simulink model "cell_EC_model"  (R2024a)
settings: Solver=VariableStepAuto  StartTime=0.0  StopTime=stop_time  FixedStep=0.5  MaxStep=.1  RelTol=1e-3
values from neighbouring files (symbols this model uses):
  C1c = data(2:end, 2:end)    [plot_RC_params.m]    (also in run_cell_sim.m)
  C1d = data(2:end, 2:end)    [plot_RC_params.m]    (also in run_cell_sim.m)
  C2c = data(2:end, 2:end)    [plot_RC_params.m]    (also in run_cell_sim.m)
  C2d = data(2:end, 2:end)    [plot_RC_params.m]    (also in run_cell_sim.m)
  C3c = data(2:end, 2:end)    [plot_RC_params.m]    (also in run_cell_sim.m)
  C3d = data(2:end, 2:end)    [plot_RC_params.m]    (also in run_cell_sim.m)
  capacity = 115.8    [extract_R0.m]    (also in identify_pulses.m; optimise_RC_parameters.m = params(7); run_cell_sim.m)
  OCV_SOC = data(2:end, 1)    [run_cell_sim.m]
  OCV_T = data(1, 2:end)    [run_cell_sim.m]
  OCV_V = data(2:end, 2:end)    [run_cell_sim.m]
  R0c = data(2:end, 2:end)    [plot_RC_params.m]    (also in run_cell_sim.m)
  R0d = data(2:end, 2:end)    [plot_RC_params.m]    (also in run_cell_sim.m)
  R1c = data(2:end, 2:end)    [plot_RC_params.m]    (also in run_cell_sim.m)
  R1d = data(2:end, 2:end)    [plot_RC_params.m]    (also in run_cell_sim.m)
  R2c = data(2:end, 2:end)    [plot_RC_params.m]    (also in run_cell_sim.m)
  R2d = data(2:end, 2:end)    [plot_RC_params.m]    (also in run_cell_sim.m)
  R3c = data(2:end, 2:end)    [plot_RC_params.m]    (also in run_cell_sim.m)
  R3d = data(2:end, 2:end)    [plot_RC_params.m]    (also in run_cell_sim.m)
  RC_SOC = data(1, 2:end)    [plot_RC_params.m]    (also in run_cell_sim.m)
  RC_T = data(2:end, 1)    [plot_RC_params.m]    (also in run_cell_sim.m)
  soc_in = interp1(OCV.V(:, find(OCV.T == temperature)), OCV.SOC, actual_voltage_full.Data(1), "linear", 'extrap')    [optimise_RC_parameters.m]    (also in run_cell_sim.m = 1)
libraries: nesl_utility x13, fl_lib x9, ee_lib x3
settings Model: Creator=mmackenzie  LastModifiedBy=mmackenzie
settings OptimizationCC: ReuseModelBlockBuffer=off
settings RTWCC: GPUComputeCapability=3.5

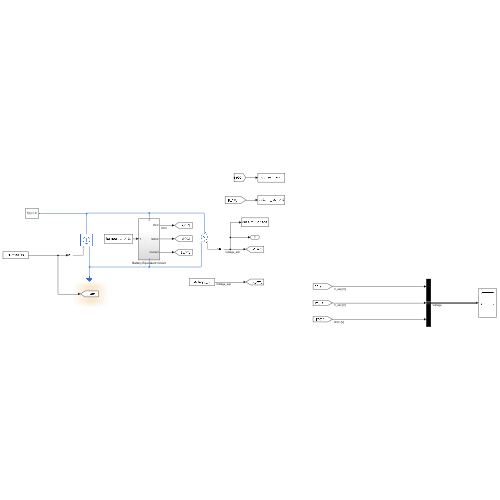
[thumbnail: Simulink's stored preview of the top-level diagram]
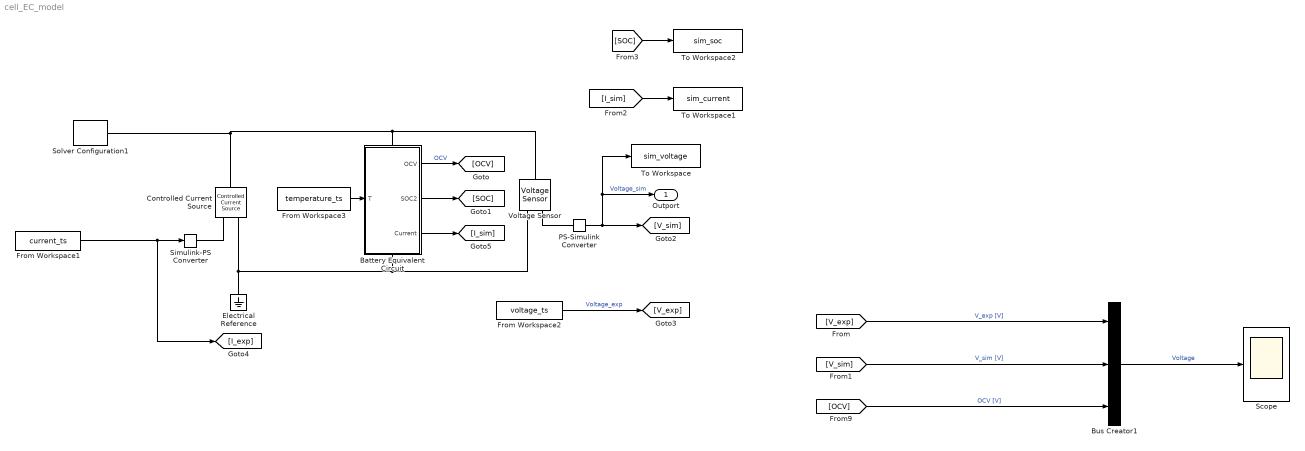
== system cell_EC_model ==
  Battery Equivalent Circuit : Subsystem
      settings: PortSchema="{\"entries\":[{\"content\":{\"sides\":[{\"content\":{\"connectorIds\":[\"In1\"]},\"type\":\"ConnectorPlacement.EquallySpacedRectSide\",\"uuid\":\"397b6d9d-31ba-4533-8816-c8a956765ed5\"},{\"content\":{\"connectorIds\":[\"Out1\",\"Out2\",\"Out3\"],\"side\":\"RIGHT\"},\"type\":\"ConnectorPlacement.EquallySpacedRectSide\",\"uuid\":\"178b2ca9-d2d9-4380-91aa-f4497cccdf4f\"},{\"content\":{\"connectorIds\":[\"LConn1\"],\"side\":\"TOP\"},\"type\":\"ConnectorPlacement.EquallySpacedRectSide\",\"uuid\":\"4710d0ae-2920-4204-9cef-cbb5eb77e7ed\"},{\"content\":{\"connectorIds\":[\"RConn1\"],\"side\":\"BOTTOM\"},\"type\":\"ConnectorPlacement.EquallySpacedRectSide\",\"uuid\":\"673921ba-ed04-43cc-8806-353dbfb62c12\"}]},\"type\":\"ConnectorPlacement.EquallySpacedConnector\",\"uuid\":\"77ff7300-8565-4430-8966-d92537bdab4b\"}],\"packageUris\":[\"http://schema.mathworks.com/mf0/Connector/R2020b\"],\"version\":\"1.0\"}"
  Bus Creator1 : BusCreator  Inputs=3
  Controlled Current Source : fl_lib/Electrical/Electrical Sources/Controlled Current Source
  Electrical Reference : fl_lib/Electrical/Electrical Elements/Electrical Reference
  From Workspace1 : FromWorkspace  VariableName=current_ts  SampleTime=-1
  From Workspace2 : FromWorkspace  VariableName=voltage_ts  SampleTime=-1
  From Workspace3 : FromWorkspace  VariableName=temperature_ts  SampleTime=-1
  PS-Simulink Converter : nesl_utility/PS-Simulink Converter  PhysicalDomain=network_engine_domain  SubClassName=ps_output  LeftPortType=input  RightPortType=output  PseudoPeriodic=off  Frequencies=[]  VectorFormat=inherit  Unit=inherit  AffineConversion=off
  Scope : Scope
  Simulink-PS Converter : nesl_utility/Simulink-PS Converter  PhysicalDomain=network_engine_domain  SubClassName=ps_input  LeftPortType=input  RightPortType=output  PseudoPeriodic=off  Frequencies=[]  NoiseDistribution=none  NoiseParameters=[]  Unit=1  AffineConversion=off  FilteringAndDerivatives=provide  SimscapeFilterOrder=1  InputFilterTimeConstant=0.001  UdotUserProvided=0
  Solver Configuration1 : nesl_utility/Solver Configuration  PhysicalDomain=network_engine_domain  SubClassName=solver  LeftPortType=input  RightPortType=generic  Tones=[]  Harmonics=[]  SimulateNoise=off  Profile=off  UseLocalSampling=off  EnableSwitchedLinearOptims=on  FrequencyDomain=off  UseCCode=off  RelTol=0.001  AbsTol=0.001  MinStep=1e-09  ToWorkspace=off  RevertToSquareIcSolve=off  NumHomotopyIterations=100  PhasorMode=off  PhasorModeNumHarmonics=1  ConsistencySolver=NEWTON_FTOL  IndexReductionMethod=DerivativeReplacement  DoDC=off  ResidualTolerance=1e-09  ConsistencyTolSource=GLOBAL  ConsistencyAbsTol=0.001  ConsistencyRelTol=0.001  ConsistencyTolFactor=0.001  UseLocalSolver=on  LocalSolverChoice=NE_BACKWARD_EULER_ADVANCER  ResolveIndetEquations=on  FunctionEvalNumThread=1  LocalSolverSampleTime=0.1  DoFixedCost=on  MaxNonlinIter=3  MaxModeIter=2  ComputeImpulses=off  ImpulseIterations=2  LinearAlgebra=auto  LinearAlgebraNumThread=0  EquationFormulation=NE_TIME_EF  DelaysMemoryBudget=1024  AutomaticFiltering=on  FilteringTimeConstant=0.001  PartitionStorageMethod=AS_NEEDED  PartitionMemoryBudget=1024  PartitionMethod=ROBUST  MultibodyUseLocalSolver=off  MultibodyLocalSolverChoice=ODE1  MultibodyLocalSolverSampleTime=0.001
  To Workspace : ToWorkspace  VariableName=sim_voltage  SampleTime=-1
      settings: Save2DSignal=2-D array (concatenate along first dimension)
  To Workspace1 : ToWorkspace  VariableName=sim_current  SaveFormat=Timeseries  SampleTime=-1
  To Workspace2 : ToWorkspace  VariableName=sim_soc  SaveFormat=Timeseries  SampleTime=-1
  Voltage Sensor : fl_lib/Electrical/Electrical Sensors/Voltage Sensor
  Outport : Outport
  wires:
  Battery Equivalent Circuit/1(OCV) -> [OCV]  "OCV"
  From Workspace2/1 -> [V_exp]  "Voltage_exp"
  PS-Simulink Converter/1 -> To Workspace/1, Outport/1, [V_sim]  "Voltage_sim"
  [V_exp] -> Bus Creator1/1  "V_exp [V]"
  Bus Creator1/1 -> Scope/1  "Voltage"
  [V_sim] -> Bus Creator1/2  "V_sim [V]"
  [OCV] -> Bus Creator1/3  "OCV [V]"
  From Workspace1/1 -> [I_exp], Simulink-PS Converter/1
  From Workspace3/1 -> Battery Equivalent Circuit/1(T)
  [I_sim] -> To Workspace1/1
  [SOC] -> To Workspace2/1
  Battery Equivalent Circuit/3(Current) -> [I_sim]
  Battery Equivalent Circuit/2(SOC2) -> [SOC]
  connections:
  Electrical Reference/LConn1 -- Voltage Sensor/RConn2 -- Battery Equivalent Circuit/RConn1 -- Controlled Current Source/RConn2
  Simulink-PS Converter/RConn1 -- Controlled Current Source/RConn1
  PS-Simulink Converter/LConn1 -- Voltage Sensor/RConn1
  Voltage Sensor/LConn1 -- Solver Configuration1/RConn1 -- Controlled Current Source/LConn1 -- Battery Equivalent Circuit/LConn1

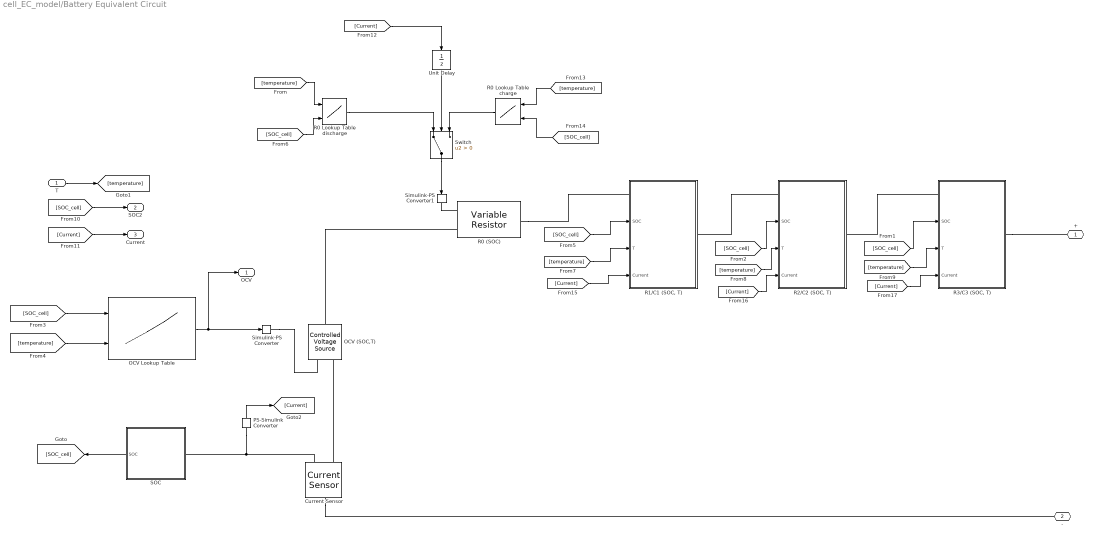
== system cell_EC_model/Battery Equivalent Circuit ==
  T : Inport
  Current Sensor : fl_lib/Electrical/Electrical Sensors/Current Sensor
  OCV (SOC,T) : fl_lib/Electrical/Electrical Sources/Controlled Voltage Source
  OCV Lookup Table : Lookup_n-D  BreakpointsForDimension1=OCV_SOC  BreakpointsForDimension2=OCV_T  Table=OCV_V  ExtrapMethod=Clip  UseLastTableValue=on  InternalRulePriority=Speed  RndMeth=Simplest
      settings: InputPortMap=u0,u1
  PS-Simulink Converter : nesl_utility/PS-Simulink Converter  PhysicalDomain=network_engine_domain  SubClassName=ps_output  LeftPortType=input  RightPortType=output  PseudoPeriodic=off  Frequencies=[]  VectorFormat=inherit  Unit=inherit  AffineConversion=off
  R0 (SOC) : fl_lib/Electrical/Electrical Elements/Variable Resistor  Rmin=0 Ohm  thermalEnable=false  thermal_mass=1 J/K  i_specify=off  i_priority=None  i=0 A  i_nominal_specify=off  i_nominal_value=1  i_nominal_unit=A  v_specify=off  v_priority=None  v=0 V  v_nominal_specify=off  v_nominal_value=1  v_nominal_unit=V  T_specify=off  T_priority=None  T=300 K  T_nominal_specify=off  T_nominal_value=1  T_nominal_unit=K
  R0 Lookup Table charge : Lookup_n-D  BreakpointsForDimension1=RC_T  BreakpointsForDimension2=RC_SOC  Table=R0c  InternalRulePriority=Speed  RndMeth=Simplest
      settings: InputPortMap=u0,u1
  R0 Lookup Table discharge : Lookup_n-D  BreakpointsForDimension1=RC_T  BreakpointsForDimension2=RC_SOC  Table=R0d  InternalRulePriority=Speed  RndMeth=Simplest
      settings: InputPortMap=u0,u1
  "R1/C1 (SOC, T)" : Subsystem
      settings: PortSchema="{\"entries\":[{\"content\":{\"sides\":[{\"content\":{\"connectorIds\":[\"LConn1\",\"In1\",\"In2\",\"In3\"]},\"type\":\"ConnectorPlacement.EquallySpacedRectSide\",\"uuid\":\"c316f4d5-4ee3-4f31-94ae-630db377ee57\"},{\"content\":{\"connectorIds\":[\"RConn1\"],\"side\":\"RIGHT\"},\"type\":\"ConnectorPlacement.EquallySpacedRectSide\",\"uuid\":\"290ce4a0-a5ae-4ffa-bce5-68eaebe420b2\"},{\"content\":{\"connectorIds\":[],\"side\":\"TOP\"},\"type\":\"ConnectorPlacement.EquallySpacedRectSide\",\"uuid\":\"08b301c6-737b-4c96-90d5-35c84b053e01\"}]},\"type\":\"ConnectorPlacement.EquallySpacedConnector\",\"uuid\":\"3d3f4144-830a-466b-8a6c-edee7622600d\"}],\"packageUris\":[\"http://schema.mathworks.com/mf0/Connector/R2020b\"],\"version\":\"1.0\"}"
  "R2/C2 (SOC, T)" : Subsystem
      settings: PortSchema="{\"entries\":[{\"content\":{\"sides\":[{\"content\":{\"connectorIds\":[\"LConn1\",\"In1\",\"In2\",\"In3\"]},\"type\":\"ConnectorPlacement.EquallySpacedRectSide\",\"uuid\":\"c316f4d5-4ee3-4f31-94ae-630db377ee57\"},{\"content\":{\"connectorIds\":[\"RConn1\"],\"side\":\"RIGHT\"},\"type\":\"ConnectorPlacement.EquallySpacedRectSide\",\"uuid\":\"290ce4a0-a5ae-4ffa-bce5-68eaebe420b2\"},{\"content\":{\"connectorIds\":[],\"side\":\"TOP\"},\"type\":\"ConnectorPlacement.EquallySpacedRectSide\",\"uuid\":\"08b301c6-737b-4c96-90d5-35c84b053e01\"}]},\"type\":\"ConnectorPlacement.EquallySpacedConnector\",\"uuid\":\"3d3f4144-830a-466b-8a6c-edee7622600d\"}],\"packageUris\":[\"http://schema.mathworks.com/mf0/Connector/R2020b\"],\"version\":\"1.0\"}"
  "R3/C3 (SOC, T)" : Subsystem
      settings: PortSchema="{\"entries\":[{\"content\":{\"sides\":[{\"content\":{\"connectorIds\":[\"LConn1\",\"In1\",\"In2\",\"In3\"]},\"type\":\"ConnectorPlacement.EquallySpacedRectSide\",\"uuid\":\"c316f4d5-4ee3-4f31-94ae-630db377ee57\"},{\"content\":{\"connectorIds\":[\"RConn1\"],\"side\":\"RIGHT\"},\"type\":\"ConnectorPlacement.EquallySpacedRectSide\",\"uuid\":\"290ce4a0-a5ae-4ffa-bce5-68eaebe420b2\"},{\"content\":{\"connectorIds\":[],\"side\":\"TOP\"},\"type\":\"ConnectorPlacement.EquallySpacedRectSide\",\"uuid\":\"08b301c6-737b-4c96-90d5-35c84b053e01\"}]},\"type\":\"ConnectorPlacement.EquallySpacedConnector\",\"uuid\":\"3d3f4144-830a-466b-8a6c-edee7622600d\"}],\"packageUris\":[\"http://schema.mathworks.com/mf0/Connector/R2020b\"],\"version\":\"1.0\"}"
  SOC : Subsystem
      settings: PortSchema="{\"entries\":[{\"content\":{\"sides\":[{\"content\":{\"connectorIds\":[\"Out1\"]},\"type\":\"ConnectorPlacement.EquallySpacedRectSide\",\"uuid\":\"7d8ebd59-8052-4308-b26c-7ff9f1f69d1b\"},{\"content\":{\"connectorIds\":[\"RConn1\"],\"side\":\"RIGHT\"},\"type\":\"ConnectorPlacement.EquallySpacedRectSide\",\"uuid\":\"c18676c0-c2b9-46af-80cc-bb3d6a3fac14\"},{\"content\":{\"connectorIds\":[],\"side\":\"TOP\"},\"type\":\"ConnectorPlacement.EquallySpacedRectSide\",\"uuid\":\"047d6f7f-9f32-4229-9b30-4a4b1fb31892\"}]},\"type\":\"ConnectorPlacement.EquallySpacedConnector\",\"uuid\":\"faef4339-4ab6-438f-b9c7-b924a206f9a5\"}],\"packageUris\":[\"http://schema.mathworks.com/mf0/Connector/R2020b\"],\"version\":\"1.0\"}"
  Simulink-PS Converter : nesl_utility/Simulink-PS Converter  PhysicalDomain=network_engine_domain  SubClassName=ps_input  LeftPortType=input  RightPortType=output  PseudoPeriodic=off  Frequencies=[]  NoiseDistribution=none  NoiseParameters=[]  Unit=1  AffineConversion=off  FilteringAndDerivatives=provide  SimscapeFilterOrder=1  InputFilterTimeConstant=0.001  UdotUserProvided=0
  Simulink-PS Converter1 : nesl_utility/Simulink-PS Converter  PhysicalDomain=network_engine_domain  SubClassName=ps_input  LeftPortType=input  RightPortType=output  PseudoPeriodic=off  Frequencies=[]  NoiseDistribution=none  NoiseParameters=[]  Unit=1  AffineConversion=off  FilteringAndDerivatives=provide  SimscapeFilterOrder=1  InputFilterTimeConstant=0.001  UdotUserProvided=0
  Switch : Switch  Criteria=u2 > Threshold  SaturateOnIntegerOverflow=off  InputSameDT=off
  Unit Delay : UnitDelay  SampleTime=-1  HasFrameUpgradeWarning=on
  + : PMIOPort  Side=Left
  - : PMIOPort  Port=2  Side=Right
  OCV : Outport
  SOC2 : Outport  Port=2
  Current : Outport  Port=3
  wires:
  SOC/1(SOC) -> [SOC_cell]
  [SOC_cell] -> OCV Lookup Table/1
  [temperature] -> OCV Lookup Table/2
  OCV Lookup Table/1 -> Simulink-PS Converter/1, OCV/1
  T/1 -> [temperature]
  [SOC_cell] -> "R3/C3 (SOC, T)"/1(SOC)
  [SOC_cell] -> "R2/C2 (SOC, T)"/1(SOC)
  [temperature] -> "R3/C3 (SOC, T)"/2(T)
  [SOC_cell] -> "R1/C1 (SOC, T)"/1(SOC)
  [temperature] -> "R2/C2 (SOC, T)"/2(T)
  [SOC_cell] -> R0 Lookup Table discharge/2
  [temperature] -> R0 Lookup Table discharge/1
  [temperature] -> "R1/C1 (SOC, T)"/2(T)
  PS-Simulink Converter/1 -> [Current]
  [SOC_cell] -> SOC2/1
  [Current] -> Current/1
  [Current] -> Unit Delay/1
  R0 Lookup Table discharge/1 -> Switch/1
  [temperature] -> R0 Lookup Table charge/1
  [SOC_cell] -> R0 Lookup Table charge/2
  R0 Lookup Table charge/1 -> Switch/3
  Switch/1 -> Simulink-PS Converter1/1
  [Current] -> "R1/C1 (SOC, T)"/3(Current)
  [Current] -> "R2/C2 (SOC, T)"/3(Current)
  [Current] -> "R3/C3 (SOC, T)"/3(Current)
  Unit Delay/1 -> Switch/2
  connections:
  Current Sensor/RConn1 -- PS-Simulink Converter/LConn1 -- SOC/RConn1
  Simulink-PS Converter/RConn1 -- OCV (SOC,T)/RConn1
  Current Sensor/LConn1 -- -/RConn1
  Current Sensor/RConn2 -- OCV (SOC,T)/RConn2
  "R3/C3 (SOC, T)"/RConn1 -- +/RConn1
  Simulink-PS Converter1/RConn1 -- R0 (SOC)/LConn1
  "R3/C3 (SOC, T)"/LConn1 -- "R2/C2 (SOC, T)"/RConn1
  "R2/C2 (SOC, T)"/LConn1 -- "R1/C1 (SOC, T)"/RConn1
  R0 (SOC)/RConn1 -- "R1/C1 (SOC, T)"/LConn1
  OCV (SOC,T)/LConn1 -- R0 (SOC)/LConn2

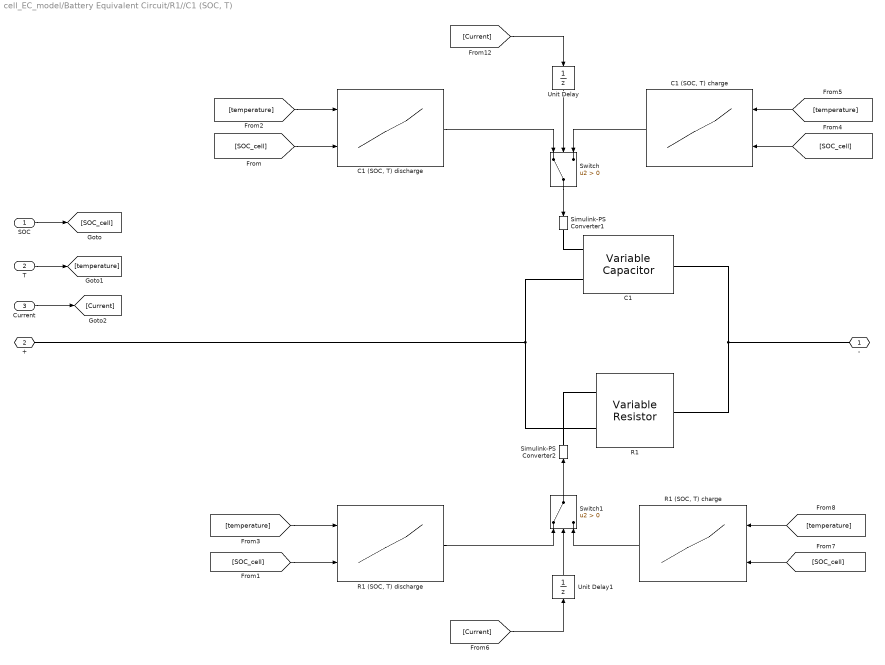
== system cell_EC_model/Battery Equivalent Circuit/R1//C1 (SOC, T) ==
  SOC : Inport
  T : Inport  Port=2
  Current : Inport  Port=3
  C1 : ee_lib/Passive/Variable Capacitor  prm=2  Cmin=1e-9 F  r=1e-6 Ohm  v0=0 V  q0=0 C
      settings: InternalSimscapePortConfiguration="{\"Bottom\":[],\"Left\":[{\"id\":\"C\",\"label\":\"C\",\"type\":\"input\"},{\"id\":\"p\",\"label\":\"+\",\"type\":\"foundation.electrical.electrical\"}],\"Right\":[{\"id\":\"n\",\"label\":\"-\",\"type\":\"foundation.electrical.electrical\"}],\"Top\":[]}"
  "C1 (SOC, T) charge" : Lookup_n-D  BreakpointsForDimension1=RC_T  BreakpointsForDimension2=RC_SOC  Table=C1c  InternalRulePriority=Speed  RndMeth=Simplest
      settings: InputPortMap=u0,u1
  "C1 (SOC, T) discharge" : Lookup_n-D  BreakpointsForDimension1=RC_T  BreakpointsForDimension2=RC_SOC  Table=C1d  InternalRulePriority=Speed  RndMeth=Simplest
      settings: InputPortMap=u0,u1
  R1 : fl_lib/Electrical/Electrical Elements/Variable Resistor  Rmin=0 Ohm  thermalEnable=false  thermal_mass=1 J/K  i_specify=off  i_priority=None  i=0 A  i_nominal_specify=off  i_nominal_value=1  i_nominal_unit=A  v_specify=off  v_priority=None  v=0 V  v_nominal_specify=off  v_nominal_value=1  v_nominal_unit=V  T_specify=off  T_priority=None  T=300 K  T_nominal_specify=off  T_nominal_value=1  T_nominal_unit=K
  "R1 (SOC, T) charge" : Lookup_n-D  BreakpointsForDimension1=RC_T  BreakpointsForDimension2=RC_SOC  Table=R1c  InternalRulePriority=Speed  RndMeth=Simplest
      settings: InputPortMap=u0,u1
  "R1 (SOC, T) discharge" : Lookup_n-D  BreakpointsForDimension1=RC_T  BreakpointsForDimension2=RC_SOC  Table=R1d  InternalRulePriority=Speed  RndMeth=Simplest
      settings: InputPortMap=u0,u1
  Simulink-PS Converter1 : nesl_utility/Simulink-PS Converter  PhysicalDomain=network_engine_domain  SubClassName=ps_input  LeftPortType=input  RightPortType=output  PseudoPeriodic=off  Frequencies=[]  NoiseDistribution=none  NoiseParameters=[]  Unit=1  AffineConversion=off  FilteringAndDerivatives=provide  SimscapeFilterOrder=1  InputFilterTimeConstant=0.001  UdotUserProvided=0
  Simulink-PS Converter2 : nesl_utility/Simulink-PS Converter  PhysicalDomain=network_engine_domain  SubClassName=ps_input  LeftPortType=input  RightPortType=output  PseudoPeriodic=off  Frequencies=[]  NoiseDistribution=none  NoiseParameters=[]  Unit=1  AffineConversion=off  FilteringAndDerivatives=provide  SimscapeFilterOrder=1  InputFilterTimeConstant=0.001  UdotUserProvided=0
  Switch : Switch  Criteria=u2 > Threshold  SaturateOnIntegerOverflow=off  InputSameDT=off
  Switch1 : Switch  Criteria=u2 > Threshold  SaturateOnIntegerOverflow=off  InputSameDT=off
  Unit Delay : UnitDelay  SampleTime=-1  HasFrameUpgradeWarning=on
  Unit Delay1 : UnitDelay  SampleTime=-1  HasFrameUpgradeWarning=on
  - : PMIOPort  Side=Right
  + : PMIOPort  Port=2  Side=Left
  wires:
  [SOC_cell] -> "C1 (SOC, T) discharge"/2
  [temperature] -> "C1 (SOC, T) discharge"/1
  [temperature] -> "R1 (SOC, T) discharge"/1
  T/1 -> [temperature]
  SOC/1 -> [SOC_cell]
  [SOC_cell] -> "R1 (SOC, T) discharge"/2
  Current/1 -> [Current]
  [Current] -> Unit Delay/1
  "C1 (SOC, T) charge"/1 -> Switch/3
  "C1 (SOC, T) discharge"/1 -> Switch/1
  Switch/1 -> Simulink-PS Converter1/1
  [temperature] -> "C1 (SOC, T) charge"/1
  [SOC_cell] -> "C1 (SOC, T) charge"/2
  [Current] -> Unit Delay1/1
  "R1 (SOC, T) discharge"/1 -> Switch1/1
  Switch1/1 -> Simulink-PS Converter2/1
  [temperature] -> "R1 (SOC, T) charge"/1
  [SOC_cell] -> "R1 (SOC, T) charge"/2
  "R1 (SOC, T) charge"/1 -> Switch1/3
  Unit Delay/1 -> Switch/2
  Unit Delay1/1 -> Switch1/2
  connections:
  Simulink-PS Converter1/RConn1 -- C1/LConn1
  Simulink-PS Converter2/RConn1 -- R1/LConn1
  C1/LConn2 -- R1/LConn2 -- +/RConn1
  C1/RConn1 -- R1/RConn1 -- -/RConn1

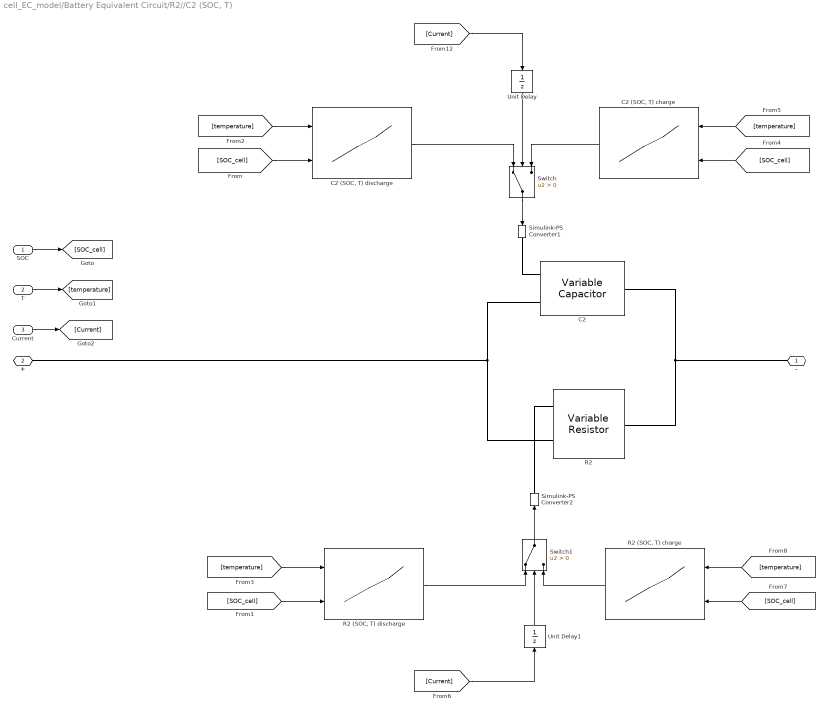
== system cell_EC_model/Battery Equivalent Circuit/R2//C2 (SOC, T) ==
  SOC : Inport
  T : Inport  Port=2
  Current : Inport  Port=3
  C2 : ee_lib/Passive/Variable Capacitor  prm=2  Cmin=1e-9 F  r=1e-6 Ohm  v0=0 V  q0=0 C
      settings: InternalSimscapePortConfiguration="{\"Bottom\":[],\"Left\":[{\"id\":\"C\",\"label\":\"C\",\"type\":\"input\"},{\"id\":\"p\",\"label\":\"+\",\"type\":\"foundation.electrical.electrical\"}],\"Right\":[{\"id\":\"n\",\"label\":\"-\",\"type\":\"foundation.electrical.electrical\"}],\"Top\":[]}"
  "C2 (SOC, T) charge" : Lookup_n-D  BreakpointsForDimension1=RC_T  BreakpointsForDimension2=RC_SOC  Table=C2c  InternalRulePriority=Speed  RndMeth=Simplest
      settings: InputPortMap=u0,u1
  "C2 (SOC, T) discharge" : Lookup_n-D  BreakpointsForDimension1=RC_T  BreakpointsForDimension2=RC_SOC  Table=C2d  InternalRulePriority=Speed  RndMeth=Simplest
      settings: InputPortMap=u0,u1
  R2 : fl_lib/Electrical/Electrical Elements/Variable Resistor  Rmin=0 Ohm  thermalEnable=false  thermal_mass=1 J/K  i_specify=off  i_priority=None  i=0 A  i_nominal_specify=off  i_nominal_value=1  i_nominal_unit=A  v_specify=off  v_priority=None  v=0 V  v_nominal_specify=off  v_nominal_value=1  v_nominal_unit=V  T_specify=off  T_priority=None  T=300 K  T_nominal_specify=off  T_nominal_value=1  T_nominal_unit=K
  "R2 (SOC, T) charge" : Lookup_n-D  BreakpointsForDimension1=RC_T  BreakpointsForDimension2=RC_SOC  Table=R2c  InternalRulePriority=Speed  RndMeth=Simplest
      settings: InputPortMap=u0,u1
  "R2 (SOC, T) discharge" : Lookup_n-D  BreakpointsForDimension1=RC_T  BreakpointsForDimension2=RC_SOC  Table=R2d  InternalRulePriority=Speed  RndMeth=Simplest
      settings: InputPortMap=u0,u1
  Simulink-PS Converter1 : nesl_utility/Simulink-PS Converter  PhysicalDomain=network_engine_domain  SubClassName=ps_input  LeftPortType=input  RightPortType=output  PseudoPeriodic=off  Frequencies=[]  NoiseDistribution=none  NoiseParameters=[]  Unit=1  AffineConversion=off  FilteringAndDerivatives=provide  SimscapeFilterOrder=1  InputFilterTimeConstant=0.001  UdotUserProvided=0
  Simulink-PS Converter2 : nesl_utility/Simulink-PS Converter  PhysicalDomain=network_engine_domain  SubClassName=ps_input  LeftPortType=input  RightPortType=output  PseudoPeriodic=off  Frequencies=[]  NoiseDistribution=none  NoiseParameters=[]  Unit=1  AffineConversion=off  FilteringAndDerivatives=provide  SimscapeFilterOrder=1  InputFilterTimeConstant=0.001  UdotUserProvided=0
  Switch : Switch  Criteria=u2 > Threshold  SaturateOnIntegerOverflow=off  InputSameDT=off
  Switch1 : Switch  Criteria=u2 > Threshold  SaturateOnIntegerOverflow=off  InputSameDT=off
  Unit Delay : UnitDelay  SampleTime=-1  HasFrameUpgradeWarning=on
  Unit Delay1 : UnitDelay  SampleTime=-1  HasFrameUpgradeWarning=on
  - : PMIOPort  Side=Right
  + : PMIOPort  Port=2  Side=Left
  wires:
  T/1 -> [temperature]
  SOC/1 -> [SOC_cell]
  [Current] -> Unit Delay/1
  [SOC_cell] -> "C2 (SOC, T) charge"/2
  "C2 (SOC, T) discharge"/1 -> Switch/1
  [temperature] -> "C2 (SOC, T) charge"/1
  [temperature] -> "C2 (SOC, T) discharge"/1
  Switch/1 -> Simulink-PS Converter1/1
  [SOC_cell] -> "C2 (SOC, T) discharge"/2
  "C2 (SOC, T) charge"/1 -> Switch/3
  Current/1 -> [Current]
  [SOC_cell] -> "R2 (SOC, T) charge"/2
  [temperature] -> "R2 (SOC, T) charge"/1
  "R2 (SOC, T) charge"/1 -> Switch1/3
  Switch1/1 -> Simulink-PS Converter2/1
  [Current] -> Unit Delay1/1
  "R2 (SOC, T) discharge"/1 -> Switch1/1
  [temperature] -> "R2 (SOC, T) discharge"/1
  [SOC_cell] -> "R2 (SOC, T) discharge"/2
  Unit Delay/1 -> Switch/2
  Unit Delay1/1 -> Switch1/2
  connections:
  C2/LConn2 -- R2/LConn2 -- +/RConn1
  C2/RConn1 -- R2/RConn1 -- -/RConn1
  Simulink-PS Converter1/RConn1 -- C2/LConn1
  Simulink-PS Converter2/RConn1 -- R2/LConn1

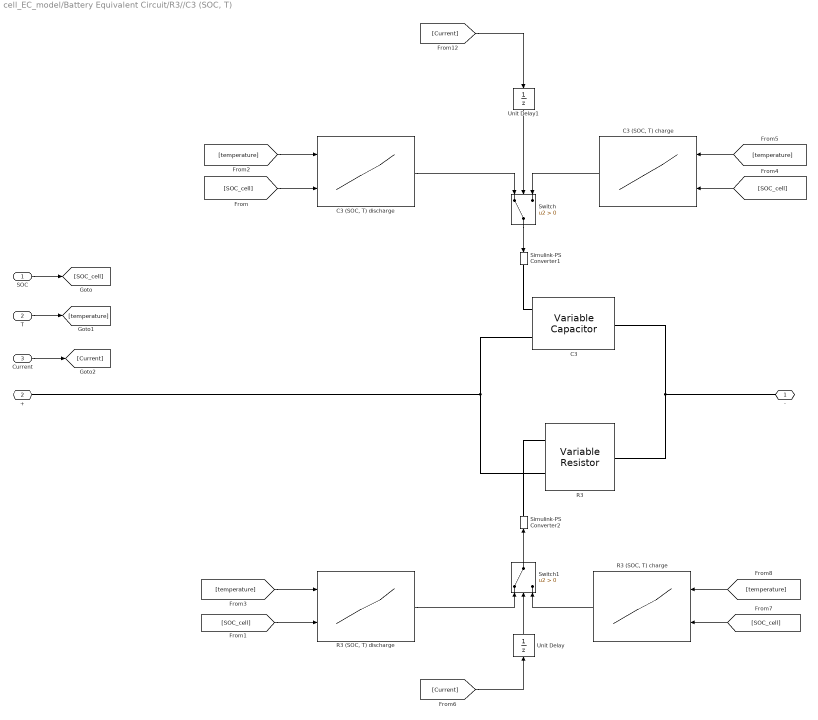
== system cell_EC_model/Battery Equivalent Circuit/R3//C3 (SOC, T) ==
  SOC : Inport
  T : Inport  Port=2
  Current : Inport  Port=3
  C3 : ee_lib/Passive/Variable Capacitor  prm=2  Cmin=1e-9 F  r=1e-6 Ohm  v0=0 V  q0=0 C
      settings: InternalSimscapePortConfiguration="{\"Bottom\":[],\"Left\":[{\"id\":\"C\",\"label\":\"C\",\"type\":\"input\"},{\"id\":\"p\",\"label\":\"+\",\"type\":\"foundation.electrical.electrical\"}],\"Right\":[{\"id\":\"n\",\"label\":\"-\",\"type\":\"foundation.electrical.electrical\"}],\"Top\":[]}"
  "C3 (SOC, T) charge" : Lookup_n-D  BreakpointsForDimension1=RC_T  BreakpointsForDimension2=RC_SOC  Table=C3c  InternalRulePriority=Speed  RndMeth=Simplest
      settings: InputPortMap=u0,u1
  "C3 (SOC, T) discharge" : Lookup_n-D  BreakpointsForDimension1=RC_T  BreakpointsForDimension2=RC_SOC  Table=C3d  InternalRulePriority=Speed  RndMeth=Simplest
      settings: InputPortMap=u0,u1
  R3 : fl_lib/Electrical/Electrical Elements/Variable Resistor  Rmin=0 Ohm  thermalEnable=false  thermal_mass=1 J/K  i_specify=off  i_priority=None  i=0 A  i_nominal_specify=off  i_nominal_value=1  i_nominal_unit=A  v_specify=off  v_priority=None  v=0 V  v_nominal_specify=off  v_nominal_value=1  v_nominal_unit=V  T_specify=off  T_priority=None  T=300 K  T_nominal_specify=off  T_nominal_value=1  T_nominal_unit=K
  "R3 (SOC, T) charge" : Lookup_n-D  BreakpointsForDimension1=RC_T  BreakpointsForDimension2=RC_SOC  Table=R3c  InternalRulePriority=Speed  RndMeth=Simplest
      settings: InputPortMap=u0,u1
  "R3 (SOC, T) discharge" : Lookup_n-D  BreakpointsForDimension1=RC_T  BreakpointsForDimension2=RC_SOC  Table=R3d  InternalRulePriority=Speed  RndMeth=Simplest
      settings: InputPortMap=u0,u1
  Simulink-PS Converter1 : nesl_utility/Simulink-PS Converter  PhysicalDomain=network_engine_domain  SubClassName=ps_input  LeftPortType=input  RightPortType=output  PseudoPeriodic=off  Frequencies=[]  NoiseDistribution=none  NoiseParameters=[]  Unit=1  AffineConversion=off  FilteringAndDerivatives=provide  SimscapeFilterOrder=1  InputFilterTimeConstant=0.001  UdotUserProvided=0
  Simulink-PS Converter2 : nesl_utility/Simulink-PS Converter  PhysicalDomain=network_engine_domain  SubClassName=ps_input  LeftPortType=input  RightPortType=output  PseudoPeriodic=off  Frequencies=[]  NoiseDistribution=none  NoiseParameters=[]  Unit=1  AffineConversion=off  FilteringAndDerivatives=provide  SimscapeFilterOrder=1  InputFilterTimeConstant=0.001  UdotUserProvided=0
  Switch : Switch  Criteria=u2 > Threshold  SaturateOnIntegerOverflow=off  InputSameDT=off
  Switch1 : Switch  Criteria=u2 > Threshold  SaturateOnIntegerOverflow=off  InputSameDT=off
  Unit Delay : UnitDelay  SampleTime=-1  HasFrameUpgradeWarning=on
  Unit Delay1 : UnitDelay  SampleTime=-1  HasFrameUpgradeWarning=on
  - : PMIOPort  Side=Right
  + : PMIOPort  Port=2  Side=Left
  wires:
  T/1 -> [temperature]
  SOC/1 -> [SOC_cell]
  [SOC_cell] -> "R3 (SOC, T) charge"/2
  [temperature] -> "R3 (SOC, T) charge"/1
  "R3 (SOC, T) charge"/1 -> Switch1/3
  Switch1/1 -> Simulink-PS Converter2/1
  [Current] -> Unit Delay/1
  "R3 (SOC, T) discharge"/1 -> Switch1/1
  [temperature] -> "R3 (SOC, T) discharge"/1
  [SOC_cell] -> "R3 (SOC, T) discharge"/2
  Current/1 -> [Current]
  [SOC_cell] -> "C3 (SOC, T) discharge"/2
  [temperature] -> "C3 (SOC, T) charge"/1
  "C3 (SOC, T) discharge"/1 -> Switch/1
  [temperature] -> "C3 (SOC, T) discharge"/1
  Switch/1 -> Simulink-PS Converter1/1
  "C3 (SOC, T) charge"/1 -> Switch/3
  [SOC_cell] -> "C3 (SOC, T) charge"/2
  [Current] -> Unit Delay1/1
  Unit Delay/1 -> Switch1/2
  Unit Delay1/1 -> Switch/2
  connections:
  C3/LConn2 -- R3/LConn2 -- +/RConn1
  C3/RConn1 -- R3/RConn1 -- -/RConn1
  Simulink-PS Converter2/RConn1 -- R3/LConn1
  C3/LConn1 -- Simulink-PS Converter1/RConn1

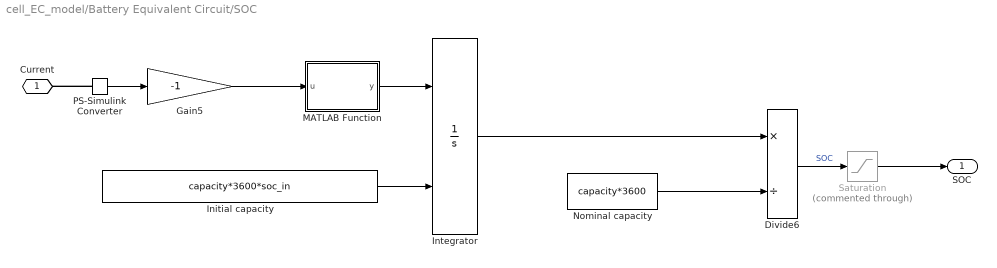
== system cell_EC_model/Battery Equivalent Circuit/SOC ==
  Divide6 : Product  Inputs=*/  RndMeth=Zero  SaturateOnIntegerOverflow=on
  Gain5 : Gain  Gain=-1
  Initial capacity : Constant  Value=capacity*3600*soc_in
  Integrator : Integrator  InitialConditionSource=external  IgnoreLimit=on  ZeroCross=off
  MATLAB Function : MATLAB Function  TreatAsAtomicUnit=on
  Nominal capacity : Constant  Value=capacity*3600
  PS-Simulink Converter : nesl_utility/PS-Simulink Converter  PhysicalDomain=network_engine_domain  SubClassName=ps_output  LeftPortType=input  RightPortType=output  PseudoPeriodic=off  Frequencies=[]  VectorFormat=inherit  Unit=inherit  AffineConversion=off
  Saturation : Saturate  Commented=through  UpperLimit=1  LowerLimit=0
  Current : PMIOPort  Side=Right
  SOC : Outport
  wires:
  Nominal capacity/1 -> Divide6/2
  Integrator/1 -> Divide6/1
  Initial capacity/1 -> Integrator/2
  Gain5/1 -> MATLAB Function/1(u)
  Divide6/1 -> Saturation/1  "SOC"
  PS-Simulink Converter/1 -> Gain5/1
  Saturation/1 -> SOC/1
  MATLAB Function/1(y) -> Integrator/1
  connections:
  PS-Simulink Converter/LConn1 -- Current/RConn1

== matlab function cell_EC_model/Battery Equivalent Circuit/SOC/MATLAB Function ==
  data: u input; y output
function y = fcn(u)
if u>0
    y=0.99*u;
else
y = u;
end
